simulink model "fuzzyPidControlDcMotor"  (R2024a)
settings: Solver=ode23tb  StartTime=0.0  StopTime=1  MaxStep=1e-5  RelTol=1e-4
libraries: spsDCMachineLib x1, spsDCVoltageSourceLib x1, spsDiodeLib x1, slpidlib x1, spsGroundLib x1, spsGtoLib x1, spsPWMGeneratorDCDCLib x1, sps_lib x1
settings Model: Creator=叉叉  LastModifiedBy=chacha
settings SolverCC: ZeroCrossControl=DisableAll  AlgebraicLoopSolver=TrustRegion
settings DebuggingCC: UnconnectedInputMsg=warning  UnconnectedOutputMsg=warning  UnconnectedLineMsg=warning
settings ModelReferenceCC: EnableRefExpFcnMdlSchedulingChecks=on
settings RTWCC: GPUComputeCapability=3.5

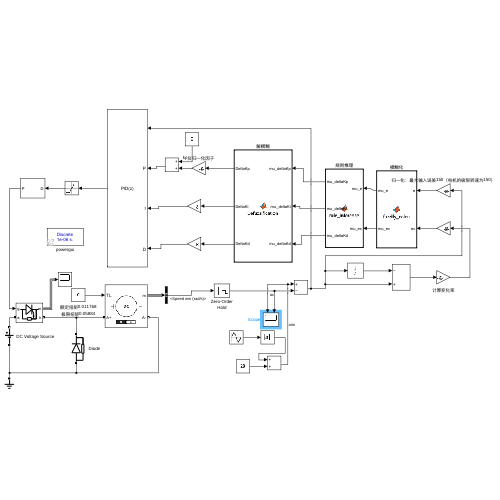
[thumbnail: Simulink's stored preview of the top-level diagram]
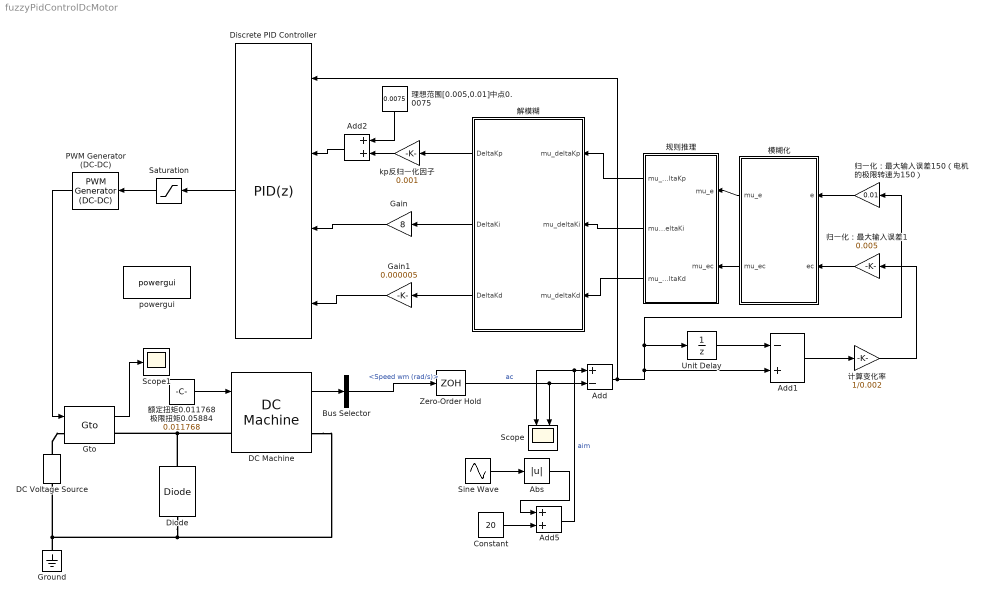
== system fuzzyPidControlDcMotor ==
  Abs : Abs  SaturateOnIntegerOverflow=off
  Add : Sum  Inputs=+-
  Add1 : Sum  Inputs=-+
  Add2 : Sum
  Add5 : Sum
  Bus Selector : BusSelector  OutputSignals=Speed wm (rad/s)
  Constant : Constant  Value=20
  DC Machine : spsDCMachineLib/DC Machine  PresetModel=No  MechanicalLoad=Torque TL  FieldType=Permanent magnet  ShowDetailedParameters=on  MeasurementBus=off  RLa="[ 7.96  0.001]"  RLf="[ 240  120]"  Laf=1.8  MachineConstant=Torque constant (N.m/A)  Ke=1.8  Kt=0.08  J=0.000001  Bm=0.000001  Tf=0.00168  w0=0  Ifinit=1  TsPowergui=0  TsBlock=-1
  DC Voltage Source : spsDCVoltageSourceLib/DC Voltage Source  Amplitude=12  Measurements=None
  Diode : spsDiodeLib/Diode  Ron=0.001  Lon=0  Vf=0.8  IC=0  UseSnubber=0  Rs=500  Cs=250e-9  Measurements=off
  Discrete PID Controller : slpidlib/PID Controller  Controller=PID  Form=Parallel  TimeDomain=Discrete-time  UseExternalTs=off  SampleTime=0.002  IntegratorMethod=Forward Euler  FilterMethod=Forward Euler  ControllerParametersSource=external  P=0.0005  I=7  UseKiTs=off  D=0.00013  UseExternalDerivativeSource=off  N=100  UseFilter=off  TunerSelectOption=Transfer Function Based (PID Tuner App)  ZeroCross=off  InitialConditionSource=internal  InitialConditionForIntegrator=0  InitialConditionForFilter=0  DifferentiatorICPrevScaledInput=0  ExternalReset=none  TrackingMode=off  Kt=1  LimitOutput=off  SatLimitsSource=internal  UpperSaturationLimit=inf  LowerSaturationLimit=-inf  LinearizeAsGain=off  AntiWindupMode=none  Kb=1  LimitIntegrator=off  UpperIntegratorSaturationLimit=inf  LowerIntegratorSaturationLimit=-inf  POutMin=[]  POutMax=[]  IOutMin=[]  IOutMax=[]  DOutMin=[]  DOutMax=[]  NOutMin=[]  NOutMax=[]  SumOutMin=[]  SumOutMax=[]  SaturationOutMin=[]  SaturationOutMax=[]  PParamMin=[]  PParamMax=[]  IParamMin=[]  IParamMax=[]  DParamMin=[]  DParamMax=[]  NParamMin=[]  NParamMax=[]  KbParamMin=[]  KbParamMax=[]  KtParamMin=[]  KtParamMax=[]  KbOutMin=[]  KbOutMax=[]  KtOutMin=[]  KtOutMax=[]  IntegratorOutMin=[]  IntegratorOutMax=[]  FilterOutMin=[]  FilterOutMax=[]  SumI1OutMin=[]  SumI1OutMax=[]  SumI2OutMin=[]  SumI2OutMax=[]  SumI3OutMin=[]  SumI3OutMax=[]  SumI4OutMin=[]  SumI4OutMax=[]  SumDOutMin=[]  SumDOutMax=[]  DifferentiatorOutMin=[]  DifferentiatorOutMax=[]  FilterDiffOutCoefMin=[]  FilterDiffOutCoefMax=[]  ReciprocalOutMin=[]  ReciprocalOutMax=[]  SumDenOutMin=[]  SumDenOutMax=[]  SumNumOutMin=[]  SumNumOutMax=[]  DivideOutMin=[]  DivideOutMax=[]  UdiffTsProdOutMin=[]  UdiffTsProdOutMax=[]  NTsProdOutMin=[]  NTsProdOutMax=[]  UintegralTsProdOutMin=[]  UintegralTsProdOutMax=[]  UngainTsProdOutMin=[]  UngainTsProdOutMax=[]  ClampingZeroOutDataTypeStr=Inherit: Inherit via back propagation  ClampingZeroOutMin=[]  ClampingZeroOutMax=[]  FilterDenConstantOutDataTypeStr=Inherit: Inherit via back propagation  FilterDenConstantOutMin=[]  FilterDenConstantOutMax=[]  PCopyOutDataTypeStr=Inherit: Inherit via back propagation  PCopyOutMin=[]  PCopyOutMax=[]  NCopyOutDataTypeStr=Inherit: Inherit via back propagation  NCopyOutMin=[]  NCopyOutMax=[]  IntegratorContinuousStateAttributes=''  IntegratorStateMustResolveToSignalObject=off  IntegratorRTWStateStorageClass=Auto  FilterContinuousStateAttributes=''  FilterStateMustResolveToSignalObject=off  FilterRTWStateStorageClass=Auto  ParallelPVariant=ExternalParameters  IdealPVariant=Disabled  IVariant=ExternalParameters  DVariant=ExternalParameters  IntegratorVariant=Discrete  SatVariant=Disabled  AWVariant=Passthrough  PCopyVariant=Disabled  TRVariant=Disabled  FdbkBlocksVariant=Forward  IdealPFdbkVariant=Disabled  SatFdbkVariant=Disabled  DerivativeFilterVariant=Differentiator  NVariant=Passthrough  NCopyVariant=Disabled_SignalSpec  FilterICVariant=InternalICsDifferentiator  IntegratorICVariant=InternalICs  ExternalResetVariant=Disabled  TRSumVariant=Passthrough  SumFdbkVariant=Disabled  SumVariant=Sum_PID  TsampFilterVariant=InternalTs  TsampNgainVariant=Passthrough  TsampIntegralVariant=Disabled_SignalSpec  ExternalSaturationOutDataTypeStr=Inherit: Same as second input  DerivativeSourceVariant=ErrorSignal
  Gain : Gain  Gain=8
  Gain1 : Gain  Gain=0.000005
  Ground : spsGroundLib/Ground  LConnTagsString=a
  Gto : spsGtoLib/Gto  Ron=0.001  Lon=0  Vf=1  Tf=10e-6  Tt=20e-6  IC=0  Rs=1e5  Cs=inf  Measurements=on
      settings: LibrarySourceBlock=sps_lib/Power Electronics/Gto
  PWM Generator (DC-DC) : spsPWMGeneratorDCDCLib/PWM Generator (DC-DC)  Fsw=5000  Ts=0
  Saturation : Saturate  UpperLimit=1  LowerLimit=0  ZeroCross=off
  Scope : Scope  NumInputPorts=2
  Scope1 : Scope
  Sine Wave : Sin  Amplitude=20  Frequency=10  SampleTime=0
  Unit Delay : UnitDelay  SampleTime=0.002  HasFrameUpgradeWarning=on
  Zero-Order Hold : ZeroOrderHold  SampleTime=0.002
  kp反归一化因子 : Gain  Gain=0.001
  powergui : sps_lib/powergui  Priority=1  SimulationMode=Discrete  SampleTime=1e-6  frequency=60  Iterations=50  frequencyindice=0  Pbase=100e6  ErrMax=1e-4  UnitsV=kV  UnitsW=MW  buscounter=0  FunctionMessages=off  echomessages=off  EnableUseOfTLC=off  CurrentSourceSwitches=off  DisableSnubberDevices=off  DisableRonSwitches=off  DisableVfSwitches=off  DisplayEquations=off  AutomaticDiscreteSolvers=off  SolverType=Tustin/Backward Euler (TBE)  Interpol=off  ExternalGateDelay=off  methode=off  Ts=100  x0status=blocks  SPID=on  SwTol=0  HookPort=off  NonlinearTolerance=1e-4  nMaxIteration=100  ContinueOnMaxIteration=off  RestoreLinks=warning  ResistiveCurrentMeasurement=off  Frange=[0:2:500]  Ylog=off  Xlog=on  ShowGrid=off  save=off  variable=ZData  structure=0  ZoomFFT=off  StartTime=0.0  cycles=1  DisplayStyle=1  fundamental=60  FreqAxis=off  MaxFrequency=1000  frequencyindicesteady=1  RmsSteady=1  display=off
  归一化：最大输入误差1 : Gain  Gain=0.005
  归一化：最大输入误差150（电机的极限转速为150） : Gain  Gain=0.01
  模糊化 : MATLAB Function  TreatAsAtomicUnit=on
  理想范围[0.005,0.01]中点0.0075 : Constant  Value=0.0075
  规则推理 : MATLAB Function  TreatAsAtomicUnit=on
  解模糊 : MATLAB Function  TreatAsAtomicUnit=on
  计算变化率 : Gain  Gain=1/0.002
  额定扭矩0.011768 极限扭矩0.05884 : Constant  Value=0.011768
  wires:
  DC Machine/1 -> Bus Selector/1
  额定扭矩0.011768 极限扭矩0.05884/1 -> DC Machine/1
  PWM Generator (DC-DC)/1 -> Gto/1
  Bus Selector/1 -> Zero-Order Hold/1  "<Speed wm (rad/s)>"
  Abs/1 -> Add5/1
  Discrete PID Controller/1 -> Saturation/1
  Saturation/1 -> PWM Generator (DC-DC)/1
  Zero-Order Hold/1 -> Add/2, Scope/2  "ac"
  模糊化/1(mu_e) -> 规则推理/1(mu_e)
  模糊化/2(mu_ec) -> 规则推理/2(mu_ec)
  Unit Delay/1 -> Add1/1
  Add1/1 -> 计算变化率/1
  Add/1 -> Add1/2, Unit Delay/1, 归一化：最大输入误差150（电机的极限转速为150）/1, Discrete PID Controller/1
  计算变化率/1 -> 归一化：最大输入误差1/1
  规则推理/2(mu_deltaKi) -> 解模糊/2(mu_deltaKi)
  规则推理/3(mu_deltaKd) -> 解模糊/3(mu_deltaKd)
  规则推理/1(mu_deltaKp) -> 解模糊/1(mu_deltaKp)
  归一化：最大输入误差1/1 -> 模糊化/2(ec)
  理想范围[0.005,0.01]中点0.0075/1 -> Add2/1
  Add2/1 -> Discrete PID Controller/2
  归一化：最大输入误差150（电机的极限转速为150）/1 -> 模糊化/1(e)
  kp反归一化因子/1 -> Add2/2
  Sine Wave/1 -> Abs/1
  解模糊/1(DeltaKp) -> kp反归一化因子/1
  Constant/1 -> Add5/2
  Add5/1 -> Scope/1, Add/1  "aim"
  解模糊/2(DeltaKi) -> Gain/1
  解模糊/3(DeltaKd) -> Gain1/1
  Gain/1 -> Discrete PID Controller/3
  Gain1/1 -> Discrete PID Controller/4
  Gto/1 -> Scope1/1
  connections:
  DC Voltage Source/RConn1 -- Gto/LConn1
  Diode/RConn1 -- DC Machine/LConn1 -- Gto/RConn1
  Diode/LConn1 -- DC Machine/RConn1 -- Ground/LConn1 -- DC Voltage Source/LConn1

== matlab function fuzzyPidControlDcMotor/规则推理 ==
  data: mu_e input; mu_deltaKp output; mu_ec input; mu_deltaKi output; mu_deltaKd output
function [mu_deltaKp, mu_deltaKi, mu_deltaKd] = rule_inference(mu_e, mu_ec)
%--------------------------------------------------
% 模糊规则推理函数
% 输入：
%   mu_e  - 误差 e 的隶属度向量 (1×7)
%   mu_ec - 误差变化率 ec 的隶属度向量 (1×7)
% 输出：
%   mu_deltaKp - ΔKp 的隶属度向量 (1×7)
%   mu_deltaKi - ΔKi 的隶属度向量 (1×7)
%   mu_deltaKd - ΔKd 的隶属度向量 (1×7)
%--------------------------------------------------

%% 1. 输出隶属度初始化（全部清零）
mu_deltaKp = zeros(1,7);   % 比例系数 Kp
mu_deltaKi = zeros(1,7);   % 积分系数 Ki
mu_deltaKd = zeros(1,7);   % 微分系数 Kd

%% 2. ΔKp 规则表（保持你原来的规则，完全不改）
% 行：误差 e
% 列：误差变化率 ec
% 数值：输出语言变量编号 (1~7)
rule_Kp = [
    7 7 6 5 4 3 2;    % e=NB: 电流反向很大，要大幅减小Kp
    6 6 5 4 3 2 2;    % e=NM
    5 5 4 3 2 2 3;    % e=NS
    4 4 3 2 2 3 4;    % e=ZO: 保持稳定
    3 2 2 3 4 5 5;    % e=PS
    2 2 3 4 5 6 6;    % e=PM
    2 3 4 5 6 7 7     % e=PB: 启动时大幅增加Kp！
];

%% 3. ΔKi 规则表（积分：小误差强，大误差弱）
rule_Ki = [
    7 7 6 6 5 4 4;
    7 6 6 5 5 4 3;
    6 6 5 5 4 3 3;
    6 5 5 4 4 3 2;
    5 5 4 4 3 2 2;
    4 4 3 3 2 2 1;
    4 3 3 2 2 1 1
];

%% 4. ΔKd 规则表（微分：变化快就增强）
rule_Kd = [
    1 2 3 4 5 6 7;
    1 2 3 4 5 6 6;
    2 3 4 5 6 6 5;
    3 4 5 6 6 5 4;
    4 5 6 6 5 4 3;
    5 6 6 5 4 3 2;
    6 6 5 4 3 2 1
];

%% 5. 模糊规则推理（Mamdani：min–max）
for i = 1:7                     % 遍历误差 e 的语言变量
    for j = 1:7                 % 遍历误差变化率 ec 的语言变量

        %--------------------------------------------------
        % 5.1 计算规则激活强度
        % 采用“与”运算 → min
        %--------------------------------------------------
        w = min(mu_e(i), mu_ec(j));

        %--------------------------------------------------
        % 5.2 Kp 推理
        %--------------------------------------------------
        lv = rule_Kp(i,j);                       % 查规则表
        mu_deltaKp(lv) = max(mu_deltaKp(lv), w); % 聚合（或运算）

        %--------------------------------------------------
        % 5.3 Ki 推理
        %--------------------------------------------------
        lv = rule_Ki(i,j);
        mu_deltaKi(lv) = max(mu_deltaKi(lv), w);

        %--------------------------------------------------
        % 5.4 Kd 推理
        %--------------------------------------------------
        lv = rule_Kd(i,j);
        mu_deltaKd(lv) = max(mu_deltaKd(lv), w);

    end
end

end

== matlab function fuzzyPidControlDcMotor/模糊化 ==
  data: e input; mu_e output; ec input; mu_ec output
function [mu_e,mu_ec] = fuzzify_calcu(e,ec)
mu_e = fuzzify(e);
mu_ec = fuzzify(ec);

== matlab function fuzzyPidControlDcMotor/解模糊 ==
  data: DeltaKp output; mu_deltaKp input; mu_deltaKi input; mu_deltaKd input; DeltaKi output; DeltaKd output
function [DeltaKp, DeltaKi, DeltaKd] = Defuzzification(mu_deltaKp, mu_deltaKi, mu_deltaKd)
% MATLAB Function 模块专用去模糊化
% 输入：
%   mu_deltaKp  - 1x7 隶属度向量
%   mu_deltaKi  - 1x7 隶属度向量
%   mu_deltaKd  - 1x7 隶属度向量
% 输出：
%   DeltaKp, DeltaKi, DeltaKd - 去模糊化数值

n_sample = 50; % 每个模糊集合采样点数

%----------------------------------------------------------
% 模糊集合顶点矩阵 [a b c]
mf = [
   -2.0   -1.5  -1.0;   % NB
   -1.0  -0.5   0.0;   % NM
   -0.5   0.0   0.5;   % NS
   -0.25  0.0   0.25;  % ZO
    0.0   0.5   1.0;   % PS
    0.5   1.0   1.5;   % PM
    1.0   1.5   2.0    % PB
];

% 去模糊化计算
DeltaKp = centroid_defuzz_safe(mu_deltaKp, mf, n_sample);
DeltaKi = centroid_defuzz_safe(mu_deltaKi, mf, n_sample);
DeltaKd = centroid_defuzz_safe(mu_deltaKd, mf, n_sample);

end

%----------------------------------------------------------
function val = centroid_defuzz_safe(mu, mf, n_sample)
% 安全的质心法去模糊化，完全避免NaN
% 输入:
%   mu - 1x7 隶属度向量
%   mf - 7x3 模糊集参数矩阵
%   n_sample - 采样点数
% 输出:
%   val - 去模糊化结果

% 1. 检查是否全零隶属度
if sum(mu) == 0
    % 返回零值（ZO的中心）
    val = 0;
    return;
end

num_mf = size(mf, 1);
val_sum = 0;
mu_sum = 0;

% 2. 对每个激活的模糊集计算
for i = 1:num_mf
    if mu(i) > 0  % 只处理激活的模糊集
        a = mf(i, 1);
        b = mf(i, 2);
        c = mf(i, 3);
        
        % 确保采样点有效
        if c <= a
            % 避免无效区间
            continue;
        end
        
        % 采样
        x = linspace(a, c, n_sample);
        
        % 计算三角形隶属度
        if abs(b - a) < eps || abs(c - b) < eps
            % 处理退化三角形（近似矩形）
            mu_tri = ones(size(x)) * mu(i);
        else
            % 正常三角形隶属度
            mu_left = (x - a) / (b - a);
            mu_right = (c - x) / (c - b);
            mu_tri = max(0, min(mu_left, mu_right));
            mu_tri = min(mu_tri, mu(i));  % Mamdani min蕴含
        end
        
        % 累加
        val_sum = val_sum + sum(x .* mu_tri);
        mu_sum = mu_sum + sum(mu_tri);
    end
end

% 3. 最终计算
if mu_sum > 0
    val = val_sum / mu_sum;
else
    % 再次检查，如果mu_sum仍然为0，返回0
    val = 0;
end

% 4. 限制在合理范围内
val = max(-2, min(2, val));

end
